simulink model "testPoly5PnP_lines_simulink"  (R2023b)
settings: Solver=FixedStepAuto  StartTime=0.0  StopTime=10.0  FixedStep=samplingTime  RelTol=1e-3
values from neighbouring files (symbols this model uses):
  pA = [1.5; 3]    [init_testPoly5PnP_lines.m]
  pB = [5; 6]    [init_testPoly5PnP_lines.m]
  pC = [5; 0]    [init_testPoly5PnP_lines.m]
  t_fAB = 4    [init_testPoly5PnP_lines.m]
  t_fBC = 8    [init_testPoly5PnP_lines.m]
  t_fCA = 9    [init_testPoly5PnP_lines.m]
  t_iAB = 1    [init_testPoly5PnP_lines.m]
settings Model: Creator=ggi01  LastModifiedBy=ggi01

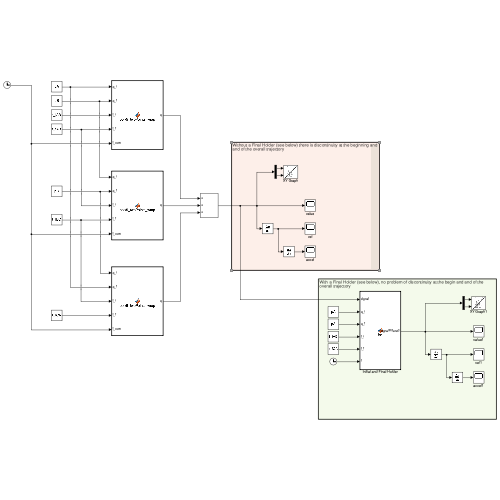
[thumbnail: Simulink's stored preview of the top-level diagram]
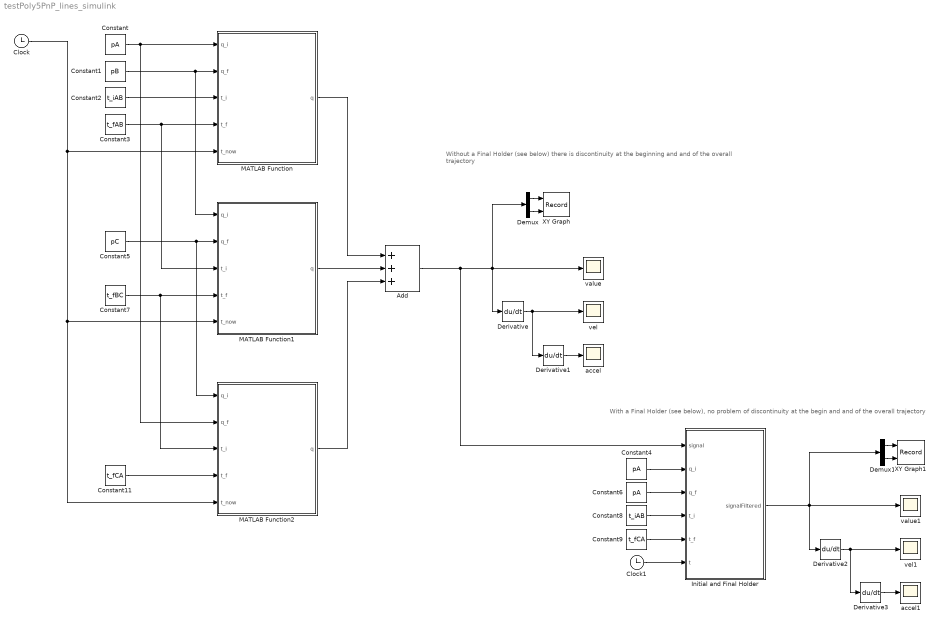
== system testPoly5PnP_lines_simulink ==
  note: Without a Final Holder (see below) there is discontinuity at the beginning and
      | and of the overall trajectory
  note: With a Final Holder (see below), no problem of discontinuity at the begin and and of the
      | overall trajectory
  Add : Sum  Inputs=+++
  Clock : Clock
  Clock1 : Clock
  Constant : Constant  Value=pA
  Constant1 : Constant  Value=pB
  Constant11 : Constant  Value=t_fCA
  Constant2 : Constant  Value=t_iAB
  Constant3 : Constant  Value=t_fAB
  Constant4 : Constant  Value=pA
  Constant5 : Constant  Value=pC
  Constant6 : Constant  Value=pA
  Constant7 : Constant  Value=t_fBC
  Constant8 : Constant  Value=t_iAB
  Constant9 : Constant  Value=t_fCA
  Demux : Demux  Outputs=2
  Demux1 : Demux  Outputs=2
  Derivative{,1..3} (4 alike) : Derivative
  Initial and Final Holder : MATLAB Function  TreatAsAtomicUnit=on
  MATLAB Function : MATLAB Function  TreatAsAtomicUnit=on
  MATLAB Function1 : MATLAB Function  TreatAsAtomicUnit=on
  MATLAB Function2 : MATLAB Function  TreatAsAtomicUnit=on
  XY Graph : Record  FileSettingsInternal="{\"entries\":[{\"content\":{\"excelSettings\":{\"content\":{},\"type\":\"Streamout.ExcelSettings\"}},\"type\":\"Streamout.FileSettingStorage\",\"uuid\":\"\"}],\"packageUris\":[\"http:\\/\\/schema.mathworks.com\\/mf0\\/streamout_blocks\\/R2020a\"],\"version\":\"1.0\"}"  Layout=[1 1]  SignalsInternal="{\"entries\":[{\"content\":{\"signals\":[{\"content\":{\"blockPath\":[],\"dimensions\":[1,1],\"domain\":\"\",\"lineColor\":\"#a2142f\",\"plots\":[ 1 ],\"port\":1,\"signalID\":1,\"signalName\":\"Demux:1\"},\"type\":\"RecordBlkView.Signal\",\"uuid\":\"\"},{\"content\":{\"blockPath\":[],\"dimensions\":[1,1],\"domain\":\"\",\"lineColor\":\"#139fff\",\"plots\":[ 1 ],\"port\":2,\"signalID\":2,\"signalName\":\"Demux:2\"},\"type\":\"RecordBlkView.Signal\",\"uuid\":\"\"}]},\"type\":\"RecordBlkView.InputSignals\",\"uuid\":\"\"}],\"packageUris\":[\"http:\\/\\/schema.mathworks.com\\/mf0\\/streamout_blocks\\/R2020a\"],\"version\":\"1.0\"}"  VisualizationBindings="{\"xyplotplugin\":{\"info\":[{\"series\":[{\"bindingParametersList\":[{\"parameter\":\"X-Axis\",\"signalID\":1,\"signalName\":\"Demux:1\"},{\"parameter\":\"Y-Axis\",\"signalID\":2,\"signalName\":\"Demux:2\"}],\"seriesID\":0}],\"subplotID\":1}]}}"  CompatibilityTag=XY
  XY Graph1 : Record  FileSettingsInternal="{\"entries\":[{\"content\":{\"excelSettings\":{\"content\":{},\"type\":\"Streamout.ExcelSettings\"}},\"type\":\"Streamout.FileSettingStorage\",\"uuid\":\"\"}],\"packageUris\":[\"http:\\/\\/schema.mathworks.com\\/mf0\\/streamout_blocks\\/R2020a\"],\"version\":\"1.0\"}"  Layout=[1 1]  SignalsInternal="{\"entries\":[{\"content\":{\"signals\":[{\"content\":{\"blockPath\":[],\"dimensions\":[1,1],\"domain\":\"\",\"lineColor\":\"#a2142f\",\"plots\":[ 1 ],\"port\":1,\"signalID\":1,\"signalName\":\"Demux1:1\"},\"type\":\"RecordBlkView.Signal\",\"uuid\":\"\"},{\"content\":{\"blockPath\":[],\"dimensions\":[1,1],\"domain\":\"\",\"lineColor\":\"#139fff\",\"plots\":[ 1 ],\"port\":2,\"signalID\":2,\"signalName\":\"Demux1:2\"},\"type\":\"RecordBlkView.Signal\",\"uuid\":\"\"}]},\"type\":\"RecordBlkView.InputSignals\",\"uuid\":\"\"}],\"packageUris\":[\"http:\\/\\/schema.mathworks.com\\/mf0\\/streamout_blocks\\/R2020a\"],\"version\":\"1.0\"}"  VisualizationBindings="{\"xyplotplugin\":{\"info\":[{\"series\":[{\"bindingParametersList\":[{\"parameter\":\"X-Axis\",\"signalID\":1,\"signalName\":\"Demux1:1\"},{\"parameter\":\"Y-Axis\",\"signalID\":2,\"signalName\":\"Demux1:2\"}],\"seriesID\":0}],\"subplotID\":1}]}}"  CompatibilityTag=XY
  accel : Scope
  accel1 : Scope
  value : Scope
  value1 : Scope
  vel : Scope
  vel1 : Scope
  wires:
  Constant/1 -> MATLAB Function2/2(q_f), MATLAB Function/1(q_i)
  Constant1/1 -> MATLAB Function1/1(q_i), MATLAB Function/2(q_f)
  Constant2/1 -> MATLAB Function/3(t_i)
  Constant3/1 -> MATLAB Function1/3(t_i), MATLAB Function/4(t_f)
  Constant7/1 -> MATLAB Function2/3(t_i), MATLAB Function1/4(t_f)
  Constant5/1 -> MATLAB Function2/1(q_i), MATLAB Function1/2(q_f)
  Constant11/1 -> MATLAB Function2/4(t_f)
  MATLAB Function/1(q) -> Add/1
  MATLAB Function2/1(q) -> Add/3
  MATLAB Function1/1(q) -> Add/2
  Add/1 -> Initial and Final Holder/1(signal), Demux/1, Derivative/1, value/1
  Clock/1 -> MATLAB Function2/5(t_now), MATLAB Function1/5(t_now), MATLAB Function/5(t_now)
  Demux/1 -> XY Graph/1
  Demux/2 -> XY Graph/2
  Derivative/1 -> Derivative1/1, vel/1
  Derivative1/1 -> accel/1
  Constant4/1 -> Initial and Final Holder/2(q_i)
  Constant6/1 -> Initial and Final Holder/3(q_f)
  Constant8/1 -> Initial and Final Holder/4(t_i)
  Constant9/1 -> Initial and Final Holder/5(t_f)
  Clock1/1 -> Initial and Final Holder/6(t)
  Demux1/1 -> XY Graph1/1
  Derivative2/1 -> Derivative3/1, vel1/1
  Initial and Final Holder/1(signalFiltered) -> Derivative2/1, Demux1/1, value1/1
  Demux1/2 -> XY Graph1/2
  Derivative3/1 -> accel1/1

== matlab function testPoly5PnP_lines_simulink/MATLAB Function1 ==
  data: q_i input; q output; q_f input; t_i input; t_f input; t_now input
function q = poly5_twoPoints_wrap(q_i, q_f, t_i, t_f, t_now)
q = poly5PnP(q_i, q_f, t_i, t_f, t_now);

== matlab function testPoly5PnP_lines_simulink/MATLAB Function ==
  data: q_i input; q output; q_f input; t_i input; t_f input; t_now input
function q = poly5_twoPoints_wrap(q_i, q_f, t_i, t_f, t_now)
q = poly5PnP(q_i, q_f, t_i, t_f, t_now);

== matlab function testPoly5PnP_lines_simulink/MATLAB Function2 ==
  data: q_i input; q output; q_f input; t_i input; t_f input; t_now input
function q = poly5_twoPoints_wrap(q_i, q_f, t_i, t_f, t_now)
q = poly5PnP(q_i, q_f, t_i, t_f, t_now);

== matlab function testPoly5PnP_lines_simulink/Initial and Final Holder ==
  data: signal input; q_i input; signalFiltered output; q_f input; t_i input; t_f input; t input
function signalFiltered = fcn(signal, q_i, q_f, t_i, t_f, t)

if t < t_i
    signalFiltered = q_i;
elseif t >= t_f
    signalFiltered = q_f;
else
    signalFiltered = signal;
end
